simulink model "feeder_1_3_ss_pmu"  (Simulink 9.2)
settings: Solver=ode4  StartTime=0.0  StopTime=inf  FixedStep=0.0001  RelTol=1e-3
PreLoadFcn:
  | Ts=100e-6;Core_Num = 0;
PostLoadFcn:
  | Ts=100e-6;Core_Num = 0;
InitFcn:
  | Ts=100e-6;Core_Num = 0;
libraries: powerlib_meascontrol x153, rtio_generic_c37_118 x17, simulink x17, artemis x2, opal_lib x2, rtlab x1, powerlib x1
(part 2 of 4)

== system feeder_1_3_ss_pmu/SS_PMU/Subsystem9 ==
  Measurements : Inport
  Demux7 : Demux  Outputs=6
  Demux8 : Demux  Outputs=6
  Mux5 : Mux  Inputs=12
  Subsystem : Subsystem
  Phasors : Outport
  Phasor_Freq : Outport  Port=2
  FROC : Outport  Port=3
  wires:
  Mux5/1 -> Phasors/1
  Demux7/4 -> [Phase_Va]
  Demux7/1 -> [Mag_Va]
  Demux7/2 -> [Mag_Vb]
  Demux7/3 -> [Mag_Vc]
  Subsystem/1(Phasors_Vabc) -> Demux7/1
  Demux7/6 -> [Phase_Vc]
  Demux7/5 -> [Phase_Vb]
  Subsystem/3(Phasor_Freq) -> Phasor_Freq/1
  Measurements/1 -> Subsystem/1(Measurements1)
  Subsystem/4(Phasor_DTFreq) -> FROC/1
  Demux8/2 -> [Mag_Ib]
  Demux8/4 -> [Phase_Ia]
  Demux8/5 -> [Phase_Ib]
  Subsystem/2(Phasors_Iabc) -> Demux8/1
  Demux8/3 -> [Mag_Ic]
  Demux8/1 -> [Mag_Ia]
  Demux8/6 -> [Phase_Ic]
  [Phase_Ic] -> Mux5/12
  [Mag_Ic] -> Mux5/11
  [Phase_Ib] -> Mux5/10
  [Mag_Ib] -> Mux5/9
  [Phase_Ia] -> Mux5/8
  [Mag_Ia] -> Mux5/7
  [Phase_Vc] -> Mux5/6
  [Mag_Vc] -> Mux5/5
  [Phase_Vb] -> Mux5/4
  [Mag_Vb] -> Mux5/3
  [Phase_Va] -> Mux5/2
  [Mag_Va] -> Mux5/1

== system feeder_1_3_ss_pmu/SS_PMU/rtlab_send_subsystem ==

== system feeder_1_3_ss_pmu/SS_PMU/zzzOpComm ==
  Demux_1 : Demux  Outputs="[102    3   14]"
  Receive_1 : opal_lib/Communication/OpRec_rt  src=1  Data_width=119  st=0.0001
  busStruct : Subsystem
  Out1 : Outport
  Out2 : Outport  Port=2
  Out3 : Outport  Port=3
  wires:
  Demux_1/3 -> busStruct/3(In3)
  Demux_1/2 -> busStruct/2(In2)
  Demux_1/1 -> busStruct/1(In1)
  busStruct/3(Out3) -> Out3/1
  busStruct/2(Out2) -> Out2/1
  busStruct/1(Out1) -> Out1/1
  Receive_1/1 -> Demux_1/1

== system feeder_1_3_ss_pmu/SS_PMU/Subsystem1/Subsystem ==
  Measurements1 : Inport
  Demux7 : Demux  Outputs=2
  Subsystem1 : Subsystem
  Phasors_Vabc : Outport
  Phasors_Iabc : Outport  Port=2
  Phasor_Freq : Outport  Port=3
  Phasor_DTFreq : Outport  Port=4
  wires:
  Measurements1/1 -> Subsystem1/1(Measurements)
  Subsystem1/2(Phasors_Freq) -> Phasor_Freq/1
  Subsystem1/3(Phasors_DTFreq) -> Phasor_DTFreq/1
  Demux7/2 -> Phasors_Iabc/1
  Demux7/1 -> Phasors_Vabc/1
  Subsystem1/1(Phasors_abc) -> Demux7/1

== system feeder_1_3_ss_pmu/SS_PMU/Subsystem10/Subsystem ==
  Measurements1 : Inport
  Demux7 : Demux  Outputs=2
  Subsystem1 : Subsystem
  Phasors_Vabc : Outport
  Phasors_Iabc : Outport  Port=2
  Phasor_Freq : Outport  Port=3
  Phasor_DTFreq : Outport  Port=4
  wires:
  Measurements1/1 -> Subsystem1/1(Measurements)
  Subsystem1/2(Phasors_Freq) -> Phasor_Freq/1
  Subsystem1/3(Phasors_DTFreq) -> Phasor_DTFreq/1
  Demux7/2 -> Phasors_Iabc/1
  Demux7/1 -> Phasors_Vabc/1
  Subsystem1/1(Phasors_abc) -> Demux7/1

== system feeder_1_3_ss_pmu/SS_PMU/Subsystem11/Subsystem ==
  Measurements1 : Inport
  Demux7 : Demux  Outputs=2
  Subsystem1 : Subsystem
  Phasors_Vabc : Outport
  Phasors_Iabc : Outport  Port=2
  Phasor_Freq : Outport  Port=3
  Phasor_DTFreq : Outport  Port=4
  wires:
  Measurements1/1 -> Subsystem1/1(Measurements)
  Subsystem1/2(Phasors_Freq) -> Phasor_Freq/1
  Subsystem1/3(Phasors_DTFreq) -> Phasor_DTFreq/1
  Demux7/2 -> Phasors_Iabc/1
  Demux7/1 -> Phasors_Vabc/1
  Subsystem1/1(Phasors_abc) -> Demux7/1

== system feeder_1_3_ss_pmu/SS_PMU/Subsystem12/Subsystem ==
  Measurements1 : Inport
  Demux7 : Demux  Outputs=2
  Subsystem1 : Subsystem
  Phasors_Vabc : Outport
  Phasors_Iabc : Outport  Port=2
  Phasor_Freq : Outport  Port=3
  Phasor_DTFreq : Outport  Port=4
  wires:
  Measurements1/1 -> Subsystem1/1(Measurements)
  Subsystem1/2(Phasors_Freq) -> Phasor_Freq/1
  Subsystem1/3(Phasors_DTFreq) -> Phasor_DTFreq/1
  Demux7/2 -> Phasors_Iabc/1
  Demux7/1 -> Phasors_Vabc/1
  Subsystem1/1(Phasors_abc) -> Demux7/1

== system feeder_1_3_ss_pmu/SS_PMU/Subsystem13/Subsystem ==
  Measurements1 : Inport
  Demux7 : Demux  Outputs=2
  Subsystem1 : Subsystem
  Phasors_Vabc : Outport
  Phasors_Iabc : Outport  Port=2
  Phasor_Freq : Outport  Port=3
  Phasor_DTFreq : Outport  Port=4
  wires:
  Measurements1/1 -> Subsystem1/1(Measurements)
  Subsystem1/2(Phasors_Freq) -> Phasor_Freq/1
  Subsystem1/3(Phasors_DTFreq) -> Phasor_DTFreq/1
  Demux7/2 -> Phasors_Iabc/1
  Demux7/1 -> Phasors_Vabc/1
  Subsystem1/1(Phasors_abc) -> Demux7/1

== system feeder_1_3_ss_pmu/SS_PMU/Subsystem14/Subsystem ==
  Measurements1 : Inport
  Demux7 : Demux  Outputs=2
  Subsystem1 : Subsystem
  Phasors_Vabc : Outport
  Phasors_Iabc : Outport  Port=2
  Phasor_Freq : Outport  Port=3
  Phasor_DTFreq : Outport  Port=4
  wires:
  Measurements1/1 -> Subsystem1/1(Measurements)
  Subsystem1/2(Phasors_Freq) -> Phasor_Freq/1
  Subsystem1/3(Phasors_DTFreq) -> Phasor_DTFreq/1
  Demux7/2 -> Phasors_Iabc/1
  Demux7/1 -> Phasors_Vabc/1
  Subsystem1/1(Phasors_abc) -> Demux7/1

== system feeder_1_3_ss_pmu/SS_PMU/Subsystem15/Subsystem ==
  Measurements1 : Inport
  Demux7 : Demux  Outputs=2
  Subsystem1 : Subsystem
  Phasors_Vabc : Outport
  Phasors_Iabc : Outport  Port=2
  Phasor_Freq : Outport  Port=3
  Phasor_DTFreq : Outport  Port=4
  wires:
  Measurements1/1 -> Subsystem1/1(Measurements)
  Subsystem1/2(Phasors_Freq) -> Phasor_Freq/1
  Subsystem1/3(Phasors_DTFreq) -> Phasor_DTFreq/1
  Demux7/2 -> Phasors_Iabc/1
  Demux7/1 -> Phasors_Vabc/1
  Subsystem1/1(Phasors_abc) -> Demux7/1

== system feeder_1_3_ss_pmu/SS_PMU/Subsystem16/Subsystem ==
  Measurements1 : Inport
  Demux7 : Demux  Outputs=2
  Subsystem1 : Subsystem
  Phasors_Vabc : Outport
  Phasors_Iabc : Outport  Port=2
  Phasor_Freq : Outport  Port=3
  Phasor_DTFreq : Outport  Port=4
  wires:
  Measurements1/1 -> Subsystem1/1(Measurements)
  Subsystem1/2(Phasors_Freq) -> Phasor_Freq/1
  Subsystem1/3(Phasors_DTFreq) -> Phasor_DTFreq/1
  Demux7/2 -> Phasors_Iabc/1
  Demux7/1 -> Phasors_Vabc/1
  Subsystem1/1(Phasors_abc) -> Demux7/1

== system feeder_1_3_ss_pmu/SS_PMU/Subsystem17/Subsystem ==
  Measurements1 : Inport
  Demux7 : Demux  Outputs=2
  Subsystem1 : Subsystem
  Phasors_Vabc : Outport
  Phasors_Iabc : Outport  Port=2
  Phasor_Freq : Outport  Port=3
  Phasor_DTFreq : Outport  Port=4
  wires:
  Measurements1/1 -> Subsystem1/1(Measurements)
  Subsystem1/2(Phasors_Freq) -> Phasor_Freq/1
  Subsystem1/3(Phasors_DTFreq) -> Phasor_DTFreq/1
  Demux7/2 -> Phasors_Iabc/1
  Demux7/1 -> Phasors_Vabc/1
  Subsystem1/1(Phasors_abc) -> Demux7/1

== system feeder_1_3_ss_pmu/SS_PMU/Subsystem2/Subsystem ==
  Measurements1 : Inport
  Demux7 : Demux  Outputs=2
  Subsystem1 : Subsystem
  Phasors_Vabc : Outport
  Phasors_Iabc : Outport  Port=2
  Phasor_Freq : Outport  Port=3
  Phasor_DTFreq : Outport  Port=4
  wires:
  Measurements1/1 -> Subsystem1/1(Measurements)
  Subsystem1/2(Phasors_Freq) -> Phasor_Freq/1
  Subsystem1/3(Phasors_DTFreq) -> Phasor_DTFreq/1
  Demux7/2 -> Phasors_Iabc/1
  Demux7/1 -> Phasors_Vabc/1
  Subsystem1/1(Phasors_abc) -> Demux7/1

== system feeder_1_3_ss_pmu/SS_PMU/Subsystem20/Subsystem ==
  In1 : Inport
  Bus Creator : BusCreator  Inputs=3
  Selector1 : Selector  InputPortWidth=14  IndexOptions=Index vector (dialog)  Indices=[13]  OutputSizes=1
  Selector2 : Selector  InputPortWidth=14  IndexOptions=Index vector (dialog)  Indices=[14]  OutputSizes=1
  Selector5 : Selector  InputPortWidth=14  IndexOptions=Index vector (dialog)  Indices=[1 2 3 4 5 6 7 8 9 10 11 12]  OutputSizes=1
  Out1 : Outport
  wires:
  In1/1 -> Selector5/1, Selector2/1, Selector1/1
  Selector5/1 -> Bus Creator/1  "Measurements"
  Bus Creator/1 -> Out1/1
  Selector1/1 -> Bus Creator/2  "FREQ"
  Selector2/1 -> Bus Creator/3  "FROC"

== system feeder_1_3_ss_pmu/SS_PMU/Subsystem21/Subsystem ==
  In1 : Inport
  Bus Creator : BusCreator  Inputs=3
  Selector1 : Selector  InputPortWidth=14  IndexOptions=Index vector (dialog)  Indices=[13]  OutputSizes=1
  Selector2 : Selector  InputPortWidth=14  IndexOptions=Index vector (dialog)  Indices=[14]  OutputSizes=1
  Selector5 : Selector  InputPortWidth=14  IndexOptions=Index vector (dialog)  Indices=[1 2 3 4 5 6 7 8 9 10 11 12]  OutputSizes=1
  Out1 : Outport
  wires:
  In1/1 -> Selector5/1, Selector2/1, Selector1/1
  Selector5/1 -> Bus Creator/1  "Measurements"
  Bus Creator/1 -> Out1/1
  Selector1/1 -> Bus Creator/2  "FREQ"
  Selector2/1 -> Bus Creator/3  "FROC"

== system feeder_1_3_ss_pmu/SS_PMU/Subsystem24/Subsystem ==
  In1 : Inport
  Bus Creator : BusCreator  Inputs=3
  Selector1 : Selector  InputPortWidth=14  IndexOptions=Index vector (dialog)  Indices=[13]  OutputSizes=1
  Selector2 : Selector  InputPortWidth=14  IndexOptions=Index vector (dialog)  Indices=[14]  OutputSizes=1
  Selector5 : Selector  InputPortWidth=14  IndexOptions=Index vector (dialog)  Indices=[1 2 3 4 5 6 7 8 9 10 11 12]  OutputSizes=1
  Out1 : Outport
  wires:
  In1/1 -> Selector5/1, Selector2/1, Selector1/1
  Selector5/1 -> Bus Creator/1  "Measurements"
  Bus Creator/1 -> Out1/1
  Selector1/1 -> Bus Creator/2  "FREQ"
  Selector2/1 -> Bus Creator/3  "FROC"

== system feeder_1_3_ss_pmu/SS_PMU/Subsystem25/Subsystem ==
  In1 : Inport
  Bus Creator : BusCreator  Inputs=3
  Selector1 : Selector  InputPortWidth=14  IndexOptions=Index vector (dialog)  Indices=[13]  OutputSizes=1
  Selector2 : Selector  InputPortWidth=14  IndexOptions=Index vector (dialog)  Indices=[14]  OutputSizes=1
  Selector5 : Selector  InputPortWidth=14  IndexOptions=Index vector (dialog)  Indices=[1 2 3 4 5 6 7 8 9 10 11 12]  OutputSizes=1
  Out1 : Outport
  wires:
  In1/1 -> Selector5/1, Selector2/1, Selector1/1
  Selector5/1 -> Bus Creator/1  "Measurements"
  Bus Creator/1 -> Out1/1
  Selector1/1 -> Bus Creator/2  "FREQ"
  Selector2/1 -> Bus Creator/3  "FROC"

== system feeder_1_3_ss_pmu/SS_PMU/Subsystem26/Subsystem ==
  In1 : Inport
  Bus Creator : BusCreator  Inputs=3
  Selector1 : Selector  InputPortWidth=14  IndexOptions=Index vector (dialog)  Indices=[13]  OutputSizes=1
  Selector2 : Selector  InputPortWidth=14  IndexOptions=Index vector (dialog)  Indices=[14]  OutputSizes=1
  Selector5 : Selector  InputPortWidth=14  IndexOptions=Index vector (dialog)  Indices=[1 2 3 4 5 6 7 8 9 10 11 12]  OutputSizes=1
  Out1 : Outport
  wires:
  In1/1 -> Selector5/1, Selector2/1, Selector1/1
  Selector5/1 -> Bus Creator/1  "Measurements"
  Bus Creator/1 -> Out1/1
  Selector1/1 -> Bus Creator/2  "FREQ"
  Selector2/1 -> Bus Creator/3  "FROC"

== system feeder_1_3_ss_pmu/SS_PMU/Subsystem27/Subsystem ==
  In1 : Inport
  Bus Creator : BusCreator  Inputs=3
  Selector1 : Selector  InputPortWidth=14  IndexOptions=Index vector (dialog)  Indices=[13]  OutputSizes=1
  Selector2 : Selector  InputPortWidth=14  IndexOptions=Index vector (dialog)  Indices=[14]  OutputSizes=1
  Selector5 : Selector  InputPortWidth=14  IndexOptions=Index vector (dialog)  Indices=[1 2 3 4 5 6 7 8 9 10 11 12]  OutputSizes=1
  Out1 : Outport
  wires:
  In1/1 -> Selector5/1, Selector2/1, Selector1/1
  Selector5/1 -> Bus Creator/1  "Measurements"
  Bus Creator/1 -> Out1/1
  Selector1/1 -> Bus Creator/2  "FREQ"
  Selector2/1 -> Bus Creator/3  "FROC"

== system feeder_1_3_ss_pmu/SS_PMU/Subsystem28/Subsystem ==
  In1 : Inport
  Bus Creator : BusCreator  Inputs=3
  Selector1 : Selector  InputPortWidth=14  IndexOptions=Index vector (dialog)  Indices=[13]  OutputSizes=1
  Selector2 : Selector  InputPortWidth=14  IndexOptions=Index vector (dialog)  Indices=[14]  OutputSizes=1
  Selector5 : Selector  InputPortWidth=14  IndexOptions=Index vector (dialog)  Indices=[1 2 3 4 5 6 7 8 9 10 11 12]  OutputSizes=1
  Out1 : Outport
  wires:
  In1/1 -> Selector5/1, Selector2/1, Selector1/1
  Selector5/1 -> Bus Creator/1  "Measurements"
  Bus Creator/1 -> Out1/1
  Selector1/1 -> Bus Creator/2  "FREQ"
  Selector2/1 -> Bus Creator/3  "FROC"

== system feeder_1_3_ss_pmu/SS_PMU/Subsystem29/Subsystem ==
  In1 : Inport
  Bus Creator : BusCreator  Inputs=3
  Selector1 : Selector  InputPortWidth=14  IndexOptions=Index vector (dialog)  Indices=[13]  OutputSizes=1
  Selector2 : Selector  InputPortWidth=14  IndexOptions=Index vector (dialog)  Indices=[14]  OutputSizes=1
  Selector5 : Selector  InputPortWidth=14  IndexOptions=Index vector (dialog)  Indices=[1 2 3 4 5 6 7 8 9 10 11 12]  OutputSizes=1
  Out1 : Outport
  wires:
  In1/1 -> Selector5/1, Selector2/1, Selector1/1
  Selector5/1 -> Bus Creator/1  "Measurements"
  Bus Creator/1 -> Out1/1
  Selector1/1 -> Bus Creator/2  "FREQ"
  Selector2/1 -> Bus Creator/3  "FROC"

== system feeder_1_3_ss_pmu/SS_PMU/Subsystem3/Subsystem ==
  Measurements1 : Inport
  Demux7 : Demux  Outputs=2
  Subsystem1 : Subsystem
  Phasors_Vabc : Outport
  Phasors_Iabc : Outport  Port=2
  Phasor_Freq : Outport  Port=3
  Phasor_DTFreq : Outport  Port=4
  wires:
  Measurements1/1 -> Subsystem1/1(Measurements)
  Subsystem1/2(Phasors_Freq) -> Phasor_Freq/1
  Subsystem1/3(Phasors_DTFreq) -> Phasor_DTFreq/1
  Demux7/2 -> Phasors_Iabc/1
  Demux7/1 -> Phasors_Vabc/1
  Subsystem1/1(Phasors_abc) -> Demux7/1

== system feeder_1_3_ss_pmu/SS_PMU/Subsystem30/Subsystem ==
  In1 : Inport
  Bus Creator : BusCreator  Inputs=3
  Selector1 : Selector  InputPortWidth=14  IndexOptions=Index vector (dialog)  Indices=[13]  OutputSizes=1
  Selector2 : Selector  InputPortWidth=14  IndexOptions=Index vector (dialog)  Indices=[14]  OutputSizes=1
  Selector5 : Selector  InputPortWidth=14  IndexOptions=Index vector (dialog)  Indices=[1 2 3 4 5 6 7 8 9 10 11 12]  OutputSizes=1
  Out1 : Outport
  wires:
  In1/1 -> Selector5/1, Selector2/1, Selector1/1
  Selector5/1 -> Bus Creator/1  "Measurements"
  Bus Creator/1 -> Out1/1
  Selector1/1 -> Bus Creator/2  "FREQ"
  Selector2/1 -> Bus Creator/3  "FROC"

== system feeder_1_3_ss_pmu/SS_PMU/Subsystem31/Subsystem ==
  In1 : Inport
  Bus Creator : BusCreator  Inputs=3
  Selector1 : Selector  InputPortWidth=14  IndexOptions=Index vector (dialog)  Indices=[13]  OutputSizes=1
  Selector2 : Selector  InputPortWidth=14  IndexOptions=Index vector (dialog)  Indices=[14]  OutputSizes=1
  Selector5 : Selector  InputPortWidth=14  IndexOptions=Index vector (dialog)  Indices=[1 2 3 4 5 6 7 8 9 10 11 12]  OutputSizes=1
  Out1 : Outport
  wires:
  In1/1 -> Selector5/1, Selector2/1, Selector1/1
  Selector5/1 -> Bus Creator/1  "Measurements"
  Bus Creator/1 -> Out1/1
  Selector1/1 -> Bus Creator/2  "FREQ"
  Selector2/1 -> Bus Creator/3  "FROC"

== system feeder_1_3_ss_pmu/SS_PMU/Subsystem32/Subsystem ==
  In1 : Inport
  Bus Creator : BusCreator  Inputs=3
  Selector1 : Selector  InputPortWidth=14  IndexOptions=Index vector (dialog)  Indices=[13]  OutputSizes=1
  Selector2 : Selector  InputPortWidth=14  IndexOptions=Index vector (dialog)  Indices=[14]  OutputSizes=1
  Selector5 : Selector  InputPortWidth=14  IndexOptions=Index vector (dialog)  Indices=[1 2 3 4 5 6 7 8 9 10 11 12]  OutputSizes=1
  Out1 : Outport
  wires:
  In1/1 -> Selector5/1, Selector2/1, Selector1/1
  Selector5/1 -> Bus Creator/1  "Measurements"
  Bus Creator/1 -> Out1/1
  Selector1/1 -> Bus Creator/2  "FREQ"
  Selector2/1 -> Bus Creator/3  "FROC"

== system feeder_1_3_ss_pmu/SS_PMU/Subsystem33/Subsystem ==
  In1 : Inport
  Bus Creator : BusCreator  Inputs=3
  Selector1 : Selector  InputPortWidth=14  IndexOptions=Index vector (dialog)  Indices=[13]  OutputSizes=1
  Selector2 : Selector  InputPortWidth=14  IndexOptions=Index vector (dialog)  Indices=[14]  OutputSizes=1
  Selector5 : Selector  InputPortWidth=14  IndexOptions=Index vector (dialog)  Indices=[1 2 3 4 5 6 7 8 9 10 11 12]  OutputSizes=1
  Out1 : Outport
  wires:
  In1/1 -> Selector5/1, Selector2/1, Selector1/1
  Selector5/1 -> Bus Creator/1  "Measurements"
  Bus Creator/1 -> Out1/1
  Selector1/1 -> Bus Creator/2  "FREQ"
  Selector2/1 -> Bus Creator/3  "FROC"

== system feeder_1_3_ss_pmu/SS_PMU/Subsystem34/Subsystem ==
  In1 : Inport
  Bus Creator : BusCreator  Inputs=3
  Selector1 : Selector  InputPortWidth=14  IndexOptions=Index vector (dialog)  Indices=[13]  OutputSizes=1
  Selector2 : Selector  InputPortWidth=14  IndexOptions=Index vector (dialog)  Indices=[14]  OutputSizes=1
  Selector5 : Selector  InputPortWidth=14  IndexOptions=Index vector (dialog)  Indices=[1 2 3 4 5 6 7 8 9 10 11 12]  OutputSizes=1
  Out1 : Outport
  wires:
  In1/1 -> Selector5/1, Selector2/1, Selector1/1
  Selector5/1 -> Bus Creator/1  "Measurements"
  Bus Creator/1 -> Out1/1
  Selector1/1 -> Bus Creator/2  "FREQ"
  Selector2/1 -> Bus Creator/3  "FROC"

== system feeder_1_3_ss_pmu/SS_PMU/Subsystem35/Subsystem ==
  In1 : Inport
  Bus Creator : BusCreator  Inputs=3
  Selector1 : Selector  InputPortWidth=14  IndexOptions=Index vector (dialog)  Indices=[13]  OutputSizes=1
  Selector2 : Selector  InputPortWidth=14  IndexOptions=Index vector (dialog)  Indices=[14]  OutputSizes=1
  Selector5 : Selector  InputPortWidth=14  IndexOptions=Index vector (dialog)  Indices=[1 2 3 4 5 6 7 8 9 10 11 12]  OutputSizes=1
  Out1 : Outport
  wires:
  In1/1 -> Selector5/1, Selector2/1, Selector1/1
  Selector5/1 -> Bus Creator/1  "Measurements"
  Bus Creator/1 -> Out1/1
  Selector1/1 -> Bus Creator/2  "FREQ"
  Selector2/1 -> Bus Creator/3  "FROC"

== system feeder_1_3_ss_pmu/SS_PMU/Subsystem36/Subsystem ==
  In1 : Inport
  Bus Creator : BusCreator  Inputs=3
  Selector1 : Selector  InputPortWidth=14  IndexOptions=Index vector (dialog)  Indices=[13]  OutputSizes=1
  Selector2 : Selector  InputPortWidth=14  IndexOptions=Index vector (dialog)  Indices=[14]  OutputSizes=1
  Selector5 : Selector  InputPortWidth=14  IndexOptions=Index vector (dialog)  Indices=[1 2 3 4 5 6 7 8 9 10 11 12]  OutputSizes=1
  Out1 : Outport
  wires:
  In1/1 -> Selector5/1, Selector2/1, Selector1/1
  Selector5/1 -> Bus Creator/1  "Measurements"
  Bus Creator/1 -> Out1/1
  Selector1/1 -> Bus Creator/2  "FREQ"
  Selector2/1 -> Bus Creator/3  "FROC"

== system feeder_1_3_ss_pmu/SS_PMU/Subsystem37/Subsystem ==
  In1 : Inport
  Bus Creator : BusCreator  Inputs=3
  Selector1 : Selector  InputPortWidth=14  IndexOptions=Index vector (dialog)  Indices=[13]  OutputSizes=1
  Selector2 : Selector  InputPortWidth=14  IndexOptions=Index vector (dialog)  Indices=[14]  OutputSizes=1
  Selector5 : Selector  InputPortWidth=14  IndexOptions=Index vector (dialog)  Indices=[1 2 3 4 5 6 7 8 9 10 11 12]  OutputSizes=1
  Out1 : Outport
  wires:
  In1/1 -> Selector5/1, Selector2/1, Selector1/1
  Selector5/1 -> Bus Creator/1  "Measurements"
  Bus Creator/1 -> Out1/1
  Selector1/1 -> Bus Creator/2  "FREQ"
  Selector2/1 -> Bus Creator/3  "FROC"

== system feeder_1_3_ss_pmu/SS_PMU/Subsystem38/Subsystem ==
  In1 : Inport
  Bus Creator : BusCreator  Inputs=3
  Selector1 : Selector  InputPortWidth=14  IndexOptions=Index vector (dialog)  Indices=[13]  OutputSizes=1
  Selector2 : Selector  InputPortWidth=14  IndexOptions=Index vector (dialog)  Indices=[14]  OutputSizes=1
  Selector5 : Selector  InputPortWidth=14  IndexOptions=Index vector (dialog)  Indices=[1 2 3 4 5 6 7 8 9 10 11 12]  OutputSizes=1
  Out1 : Outport
  wires:
  In1/1 -> Selector5/1, Selector2/1, Selector1/1
  Selector5/1 -> Bus Creator/1  "Measurements"
  Bus Creator/1 -> Out1/1
  Selector1/1 -> Bus Creator/2  "FREQ"
  Selector2/1 -> Bus Creator/3  "FROC"

== system feeder_1_3_ss_pmu/SS_PMU/Subsystem4/Subsystem ==
  Measurements1 : Inport
  Demux7 : Demux  Outputs=2
  Subsystem1 : Subsystem
  Phasors_Vabc : Outport
  Phasors_Iabc : Outport  Port=2
  Phasor_Freq : Outport  Port=3
  Phasor_DTFreq : Outport  Port=4
  wires:
  Measurements1/1 -> Subsystem1/1(Measurements)
  Subsystem1/2(Phasors_Freq) -> Phasor_Freq/1
  Subsystem1/3(Phasors_DTFreq) -> Phasor_DTFreq/1
  Demux7/2 -> Phasors_Iabc/1
  Demux7/1 -> Phasors_Vabc/1
  Subsystem1/1(Phasors_abc) -> Demux7/1

== system feeder_1_3_ss_pmu/SS_PMU/Subsystem5/Subsystem ==
  Measurements1 : Inport
  Demux7 : Demux  Outputs=2
  Subsystem1 : Subsystem
  Phasors_Vabc : Outport
  Phasors_Iabc : Outport  Port=2
  Phasor_Freq : Outport  Port=3
  Phasor_DTFreq : Outport  Port=4
  wires:
  Measurements1/1 -> Subsystem1/1(Measurements)
  Subsystem1/2(Phasors_Freq) -> Phasor_Freq/1
  Subsystem1/3(Phasors_DTFreq) -> Phasor_DTFreq/1
  Demux7/2 -> Phasors_Iabc/1
  Demux7/1 -> Phasors_Vabc/1
  Subsystem1/1(Phasors_abc) -> Demux7/1

== system feeder_1_3_ss_pmu/SS_PMU/Subsystem6/Subsystem ==
  Measurements1 : Inport
  Demux7 : Demux  Outputs=2
  Subsystem1 : Subsystem
  Phasors_Vabc : Outport
  Phasors_Iabc : Outport  Port=2
  Phasor_Freq : Outport  Port=3
  Phasor_DTFreq : Outport  Port=4
  wires:
  Measurements1/1 -> Subsystem1/1(Measurements)
  Subsystem1/2(Phasors_Freq) -> Phasor_Freq/1
  Subsystem1/3(Phasors_DTFreq) -> Phasor_DTFreq/1
  Demux7/2 -> Phasors_Iabc/1
  Demux7/1 -> Phasors_Vabc/1
  Subsystem1/1(Phasors_abc) -> Demux7/1

== system feeder_1_3_ss_pmu/SS_PMU/Subsystem7/Subsystem ==
  Measurements1 : Inport
  Demux7 : Demux  Outputs=2
  Subsystem1 : Subsystem
  Phasors_Vabc : Outport
  Phasors_Iabc : Outport  Port=2
  Phasor_Freq : Outport  Port=3
  Phasor_DTFreq : Outport  Port=4
  wires:
  Measurements1/1 -> Subsystem1/1(Measurements)
  Subsystem1/2(Phasors_Freq) -> Phasor_Freq/1
  Subsystem1/3(Phasors_DTFreq) -> Phasor_DTFreq/1
  Demux7/2 -> Phasors_Iabc/1
  Demux7/1 -> Phasors_Vabc/1
  Subsystem1/1(Phasors_abc) -> Demux7/1

== system feeder_1_3_ss_pmu/SS_PMU/Subsystem8/Subsystem ==
  Measurements1 : Inport
  Demux7 : Demux  Outputs=2
  Subsystem1 : Subsystem
  Phasors_Vabc : Outport
  Phasors_Iabc : Outport  Port=2
  Phasor_Freq : Outport  Port=3
  Phasor_DTFreq : Outport  Port=4
  wires:
  Measurements1/1 -> Subsystem1/1(Measurements)
  Subsystem1/2(Phasors_Freq) -> Phasor_Freq/1
  Subsystem1/3(Phasors_DTFreq) -> Phasor_DTFreq/1
  Demux7/2 -> Phasors_Iabc/1
  Demux7/1 -> Phasors_Vabc/1
  Subsystem1/1(Phasors_abc) -> Demux7/1

== system feeder_1_3_ss_pmu/SS_PMU/Subsystem9/Subsystem ==
  Measurements1 : Inport
  Demux7 : Demux  Outputs=2
  Subsystem1 : Subsystem
  Phasors_Vabc : Outport
  Phasors_Iabc : Outport  Port=2
  Phasor_Freq : Outport  Port=3
  Phasor_DTFreq : Outport  Port=4
  wires:
  Measurements1/1 -> Subsystem1/1(Measurements)
  Subsystem1/2(Phasors_Freq) -> Phasor_Freq/1
  Subsystem1/3(Phasors_DTFreq) -> Phasor_DTFreq/1
  Demux7/2 -> Phasors_Iabc/1
  Demux7/1 -> Phasors_Vabc/1
  Subsystem1/1(Phasors_abc) -> Demux7/1

== system feeder_1_3_ss_pmu/SS_PMU/zzzOpComm/busStruct ==
  In1 : Inport
  In2 : Inport  Port=2
  In3 : Inport  Port=3
  Sub1 : Subsystem
  Sub2 : Subsystem
  Sub3 : Subsystem
  Out1 : Outport
  Out2 : Outport  Port=2
  Out3 : Outport  Port=3
  wires:
  Sub3/1(out) -> Out3/1
  In3/1 -> Sub3/1(in)
  Sub2/1(out) -> Out2/1
  In2/1 -> Sub2/1(in)
  Sub1/1(goto_signal1) -> Out1/1
  In1/1 -> Sub1/1(from_signal1)

== system feeder_1_3_ss_pmu/SS_PMU/Subsystem1/Subsystem/Subsystem1 ==
  Measurements : Inport
  Degree to radian1 : Subsystem
  Mux1 : Mux
  Selector5 : Selector  InputPortWidth=12  IndexOptions=Index vector (dialog)  Indices=[1 3 5]  OutputSizes=1
  Selector6 : Selector  InputPortWidth=12  IndexOptions=Index vector (dialog)  Indices=[7 9 11]  OutputSizes=1
  Selector7 : Selector  InputPortWidth=6  IndexOptions=Index vector (dialog)  Indices=[1 2 3]  OutputSizes=1
  Selector8 : Selector  InputPortWidth=6  IndexOptions=Index vector (dialog)  Indices=[4 5 6]  OutputSizes=1
  Selector9 : Selector  InputPortWidth=12  IndexOptions=Index vector (dialog)  Indices=[2 4 6 8 10 12]  OutputSizes=1
  Subsystem : Subsystem
  Phasors_abc : Outport
  Phasors_Freq : Outport  Port=2
  Phasors_DTFreq : Outport  Port=3
  wires:
  Subsystem/2(Phasors_freq) -> Phasors_Freq/1
  Subsystem/3(Phasors_dtfreq1) -> Phasors_DTFreq/1
  Selector5/1 -> Mux1/1
  Mux1/1 -> Phasors_abc/1
  Selector7/1 -> Mux1/2
  Subsystem/1(Phasors_60Hz) -> Selector5/1, Selector6/1, Selector9/1
  Selector8/1 -> Mux1/4
  Selector6/1 -> Mux1/3
  Measurements/1 -> Subsystem/1(Measurements1)
  Selector9/1 -> Degree to radian1/1(Degree)
  Degree to radian1/1(Radian) -> Selector7/1, Selector8/1

== system feeder_1_3_ss_pmu/SS_PMU/Subsystem10/Subsystem/Subsystem1 ==
  Measurements : Inport
  Degree to radian1 : Subsystem
  Mux1 : Mux
  Selector5 : Selector  InputPortWidth=12  IndexOptions=Index vector (dialog)  Indices=[1 3 5]  OutputSizes=1
  Selector6 : Selector  InputPortWidth=12  IndexOptions=Index vector (dialog)  Indices=[7 9 11]  OutputSizes=1
  Selector7 : Selector  InputPortWidth=6  IndexOptions=Index vector (dialog)  Indices=[1 2 3]  OutputSizes=1
  Selector8 : Selector  InputPortWidth=6  IndexOptions=Index vector (dialog)  Indices=[4 5 6]  OutputSizes=1
  Selector9 : Selector  InputPortWidth=12  IndexOptions=Index vector (dialog)  Indices=[2 4 6 8 10 12]  OutputSizes=1
  Subsystem : Subsystem
  Phasors_abc : Outport
  Phasors_Freq : Outport  Port=2
  Phasors_DTFreq : Outport  Port=3
  wires:
  Subsystem/2(Phasors_freq) -> Phasors_Freq/1
  Subsystem/3(Phasors_dtfreq1) -> Phasors_DTFreq/1
  Selector5/1 -> Mux1/1
  Mux1/1 -> Phasors_abc/1
  Selector7/1 -> Mux1/2
  Subsystem/1(Phasors_60Hz) -> Selector5/1, Selector6/1, Selector9/1
  Selector8/1 -> Mux1/4
  Selector6/1 -> Mux1/3
  Measurements/1 -> Subsystem/1(Measurements1)
  Selector9/1 -> Degree to radian1/1(Degree)
  Degree to radian1/1(Radian) -> Selector7/1, Selector8/1

== system feeder_1_3_ss_pmu/SS_PMU/Subsystem11/Subsystem/Subsystem1 ==
  Measurements : Inport
  Degree to radian1 : Subsystem
  Mux1 : Mux
  Selector5 : Selector  InputPortWidth=12  IndexOptions=Index vector (dialog)  Indices=[1 3 5]  OutputSizes=1
  Selector6 : Selector  InputPortWidth=12  IndexOptions=Index vector (dialog)  Indices=[7 9 11]  OutputSizes=1
  Selector7 : Selector  InputPortWidth=6  IndexOptions=Index vector (dialog)  Indices=[1 2 3]  OutputSizes=1
  Selector8 : Selector  InputPortWidth=6  IndexOptions=Index vector (dialog)  Indices=[4 5 6]  OutputSizes=1
  Selector9 : Selector  InputPortWidth=12  IndexOptions=Index vector (dialog)  Indices=[2 4 6 8 10 12]  OutputSizes=1
  Subsystem : Subsystem
  Phasors_abc : Outport
  Phasors_Freq : Outport  Port=2
  Phasors_DTFreq : Outport  Port=3
  wires:
  Subsystem/2(Phasors_freq) -> Phasors_Freq/1
  Subsystem/3(Phasors_dtfreq1) -> Phasors_DTFreq/1
  Selector5/1 -> Mux1/1
  Mux1/1 -> Phasors_abc/1
  Selector7/1 -> Mux1/2
  Subsystem/1(Phasors_60Hz) -> Selector5/1, Selector6/1, Selector9/1
  Selector8/1 -> Mux1/4
  Selector6/1 -> Mux1/3
  Measurements/1 -> Subsystem/1(Measurements1)
  Selector9/1 -> Degree to radian1/1(Degree)
  Degree to radian1/1(Radian) -> Selector7/1, Selector8/1

== system feeder_1_3_ss_pmu/SS_PMU/Subsystem12/Subsystem/Subsystem1 ==
  Measurements : Inport
  Degree to radian1 : Subsystem
  Mux1 : Mux
  Selector5 : Selector  InputPortWidth=12  IndexOptions=Index vector (dialog)  Indices=[1 3 5]  OutputSizes=1
  Selector6 : Selector  InputPortWidth=12  IndexOptions=Index vector (dialog)  Indices=[7 9 11]  OutputSizes=1
  Selector7 : Selector  InputPortWidth=6  IndexOptions=Index vector (dialog)  Indices=[1 2 3]  OutputSizes=1
  Selector8 : Selector  InputPortWidth=6  IndexOptions=Index vector (dialog)  Indices=[4 5 6]  OutputSizes=1
  Selector9 : Selector  InputPortWidth=12  IndexOptions=Index vector (dialog)  Indices=[2 4 6 8 10 12]  OutputSizes=1
  Subsystem : Subsystem
  Phasors_abc : Outport
  Phasors_Freq : Outport  Port=2
  Phasors_DTFreq : Outport  Port=3
  wires:
  Subsystem/2(Phasors_freq) -> Phasors_Freq/1
  Subsystem/3(Phasors_dtfreq1) -> Phasors_DTFreq/1
  Selector5/1 -> Mux1/1
  Mux1/1 -> Phasors_abc/1
  Selector7/1 -> Mux1/2
  Subsystem/1(Phasors_60Hz) -> Selector5/1, Selector6/1, Selector9/1
  Selector8/1 -> Mux1/4
  Selector6/1 -> Mux1/3
  Measurements/1 -> Subsystem/1(Measurements1)
  Selector9/1 -> Degree to radian1/1(Degree)
  Degree to radian1/1(Radian) -> Selector7/1, Selector8/1

== system feeder_1_3_ss_pmu/SS_PMU/Subsystem13/Subsystem/Subsystem1 ==
  Measurements : Inport
  Degree to radian1 : Subsystem
  Mux1 : Mux
  Selector5 : Selector  InputPortWidth=12  IndexOptions=Index vector (dialog)  Indices=[1 3 5]  OutputSizes=1
  Selector6 : Selector  InputPortWidth=12  IndexOptions=Index vector (dialog)  Indices=[7 9 11]  OutputSizes=1
  Selector7 : Selector  InputPortWidth=6  IndexOptions=Index vector (dialog)  Indices=[1 2 3]  OutputSizes=1
  Selector8 : Selector  InputPortWidth=6  IndexOptions=Index vector (dialog)  Indices=[4 5 6]  OutputSizes=1
  Selector9 : Selector  InputPortWidth=12  IndexOptions=Index vector (dialog)  Indices=[2 4 6 8 10 12]  OutputSizes=1
  Subsystem : Subsystem
  Phasors_abc : Outport
  Phasors_Freq : Outport  Port=2
  Phasors_DTFreq : Outport  Port=3
  wires:
  Subsystem/2(Phasors_freq) -> Phasors_Freq/1
  Subsystem/3(Phasors_dtfreq1) -> Phasors_DTFreq/1
  Selector5/1 -> Mux1/1
  Mux1/1 -> Phasors_abc/1
  Selector7/1 -> Mux1/2
  Subsystem/1(Phasors_60Hz) -> Selector5/1, Selector6/1, Selector9/1
  Selector8/1 -> Mux1/4
  Selector6/1 -> Mux1/3
  Measurements/1 -> Subsystem/1(Measurements1)
  Selector9/1 -> Degree to radian1/1(Degree)
  Degree to radian1/1(Radian) -> Selector7/1, Selector8/1

== system feeder_1_3_ss_pmu/SS_PMU/Subsystem14/Subsystem/Subsystem1 ==
  Measurements : Inport
  Degree to radian1 : Subsystem
  Mux1 : Mux
  Selector5 : Selector  InputPortWidth=12  IndexOptions=Index vector (dialog)  Indices=[1 3 5]  OutputSizes=1
  Selector6 : Selector  InputPortWidth=12  IndexOptions=Index vector (dialog)  Indices=[7 9 11]  OutputSizes=1
  Selector7 : Selector  InputPortWidth=6  IndexOptions=Index vector (dialog)  Indices=[1 2 3]  OutputSizes=1
  Selector8 : Selector  InputPortWidth=6  IndexOptions=Index vector (dialog)  Indices=[4 5 6]  OutputSizes=1
  Selector9 : Selector  InputPortWidth=12  IndexOptions=Index vector (dialog)  Indices=[2 4 6 8 10 12]  OutputSizes=1
  Subsystem : Subsystem
  Phasors_abc : Outport
  Phasors_Freq : Outport  Port=2
  Phasors_DTFreq : Outport  Port=3
  wires:
  Subsystem/2(Phasors_freq) -> Phasors_Freq/1
  Subsystem/3(Phasors_dtfreq1) -> Phasors_DTFreq/1
  Selector5/1 -> Mux1/1
  Mux1/1 -> Phasors_abc/1
  Selector7/1 -> Mux1/2
  Subsystem/1(Phasors_60Hz) -> Selector5/1, Selector6/1, Selector9/1
  Selector8/1 -> Mux1/4
  Selector6/1 -> Mux1/3
  Measurements/1 -> Subsystem/1(Measurements1)
  Selector9/1 -> Degree to radian1/1(Degree)
  Degree to radian1/1(Radian) -> Selector7/1, Selector8/1

== system feeder_1_3_ss_pmu/SS_PMU/Subsystem15/Subsystem/Subsystem1 ==
  Measurements : Inport
  Degree to radian1 : Subsystem
  Mux1 : Mux
  Selector5 : Selector  InputPortWidth=12  IndexOptions=Index vector (dialog)  Indices=[1 3 5]  OutputSizes=1
  Selector6 : Selector  InputPortWidth=12  IndexOptions=Index vector (dialog)  Indices=[7 9 11]  OutputSizes=1
  Selector7 : Selector  InputPortWidth=6  IndexOptions=Index vector (dialog)  Indices=[1 2 3]  OutputSizes=1
  Selector8 : Selector  InputPortWidth=6  IndexOptions=Index vector (dialog)  Indices=[4 5 6]  OutputSizes=1
  Selector9 : Selector  InputPortWidth=12  IndexOptions=Index vector (dialog)  Indices=[2 4 6 8 10 12]  OutputSizes=1
  Subsystem : Subsystem
  Phasors_abc : Outport
  Phasors_Freq : Outport  Port=2
  Phasors_DTFreq : Outport  Port=3
  wires:
  Subsystem/2(Phasors_freq) -> Phasors_Freq/1
  Subsystem/3(Phasors_dtfreq1) -> Phasors_DTFreq/1
  Selector5/1 -> Mux1/1
  Mux1/1 -> Phasors_abc/1
  Selector7/1 -> Mux1/2
  Subsystem/1(Phasors_60Hz) -> Selector5/1, Selector6/1, Selector9/1
  Selector8/1 -> Mux1/4
  Selector6/1 -> Mux1/3
  Measurements/1 -> Subsystem/1(Measurements1)
  Selector9/1 -> Degree to radian1/1(Degree)
  Degree to radian1/1(Radian) -> Selector7/1, Selector8/1

== system feeder_1_3_ss_pmu/SS_PMU/Subsystem16/Subsystem/Subsystem1 ==
  Measurements : Inport
  Degree to radian1 : Subsystem
  Mux1 : Mux
  Selector5 : Selector  InputPortWidth=12  IndexOptions=Index vector (dialog)  Indices=[1 3 5]  OutputSizes=1
  Selector6 : Selector  InputPortWidth=12  IndexOptions=Index vector (dialog)  Indices=[7 9 11]  OutputSizes=1
  Selector7 : Selector  InputPortWidth=6  IndexOptions=Index vector (dialog)  Indices=[1 2 3]  OutputSizes=1
  Selector8 : Selector  InputPortWidth=6  IndexOptions=Index vector (dialog)  Indices=[4 5 6]  OutputSizes=1
  Selector9 : Selector  InputPortWidth=12  IndexOptions=Index vector (dialog)  Indices=[2 4 6 8 10 12]  OutputSizes=1
  Subsystem : Subsystem
  Phasors_abc : Outport
  Phasors_Freq : Outport  Port=2
  Phasors_DTFreq : Outport  Port=3
  wires:
  Subsystem/2(Phasors_freq) -> Phasors_Freq/1
  Subsystem/3(Phasors_dtfreq1) -> Phasors_DTFreq/1
  Selector5/1 -> Mux1/1
  Mux1/1 -> Phasors_abc/1
  Selector7/1 -> Mux1/2
  Subsystem/1(Phasors_60Hz) -> Selector5/1, Selector6/1, Selector9/1
  Selector8/1 -> Mux1/4
  Selector6/1 -> Mux1/3
  Measurements/1 -> Subsystem/1(Measurements1)
  Selector9/1 -> Degree to radian1/1(Degree)
  Degree to radian1/1(Radian) -> Selector7/1, Selector8/1

== system feeder_1_3_ss_pmu/SS_PMU/Subsystem17/Subsystem/Subsystem1 ==
  Measurements : Inport
  Degree to radian1 : Subsystem
  Mux1 : Mux
  Selector5 : Selector  InputPortWidth=12  IndexOptions=Index vector (dialog)  Indices=[1 3 5]  OutputSizes=1
  Selector6 : Selector  InputPortWidth=12  IndexOptions=Index vector (dialog)  Indices=[7 9 11]  OutputSizes=1
  Selector7 : Selector  InputPortWidth=6  IndexOptions=Index vector (dialog)  Indices=[1 2 3]  OutputSizes=1
  Selector8 : Selector  InputPortWidth=6  IndexOptions=Index vector (dialog)  Indices=[4 5 6]  OutputSizes=1
  Selector9 : Selector  InputPortWidth=12  IndexOptions=Index vector (dialog)  Indices=[2 4 6 8 10 12]  OutputSizes=1
  Subsystem : Subsystem
  Phasors_abc : Outport
  Phasors_Freq : Outport  Port=2
  Phasors_DTFreq : Outport  Port=3
  wires:
  Subsystem/2(Phasors_freq) -> Phasors_Freq/1
  Subsystem/3(Phasors_dtfreq1) -> Phasors_DTFreq/1
  Selector5/1 -> Mux1/1
  Mux1/1 -> Phasors_abc/1
  Selector7/1 -> Mux1/2
  Subsystem/1(Phasors_60Hz) -> Selector5/1, Selector6/1, Selector9/1
  Selector8/1 -> Mux1/4
  Selector6/1 -> Mux1/3
  Measurements/1 -> Subsystem/1(Measurements1)
  Selector9/1 -> Degree to radian1/1(Degree)
  Degree to radian1/1(Radian) -> Selector7/1, Selector8/1

== system feeder_1_3_ss_pmu/SS_PMU/Subsystem2/Subsystem/Subsystem1 ==
  Measurements : Inport
  Degree to radian1 : Subsystem
  Mux1 : Mux
  Selector5 : Selector  InputPortWidth=12  IndexOptions=Index vector (dialog)  Indices=[1 3 5]  OutputSizes=1
  Selector6 : Selector  InputPortWidth=12  IndexOptions=Index vector (dialog)  Indices=[7 9 11]  OutputSizes=1
  Selector7 : Selector  InputPortWidth=6  IndexOptions=Index vector (dialog)  Indices=[1 2 3]  OutputSizes=1
  Selector8 : Selector  InputPortWidth=6  IndexOptions=Index vector (dialog)  Indices=[4 5 6]  OutputSizes=1
  Selector9 : Selector  InputPortWidth=12  IndexOptions=Index vector (dialog)  Indices=[2 4 6 8 10 12]  OutputSizes=1
  Subsystem : Subsystem
  Phasors_abc : Outport
  Phasors_Freq : Outport  Port=2
  Phasors_DTFreq : Outport  Port=3
  wires:
  Subsystem/2(Phasors_freq) -> Phasors_Freq/1
  Subsystem/3(Phasors_dtfreq1) -> Phasors_DTFreq/1
  Selector5/1 -> Mux1/1
  Mux1/1 -> Phasors_abc/1
  Selector7/1 -> Mux1/2
  Subsystem/1(Phasors_60Hz) -> Selector5/1, Selector6/1, Selector9/1
  Selector8/1 -> Mux1/4
  Selector6/1 -> Mux1/3
  Measurements/1 -> Subsystem/1(Measurements1)
  Selector9/1 -> Degree to radian1/1(Degree)
  Degree to radian1/1(Radian) -> Selector7/1, Selector8/1

== system feeder_1_3_ss_pmu/SS_PMU/Subsystem3/Subsystem/Subsystem1 ==
  Measurements : Inport
  Degree to radian1 : Subsystem
  Mux1 : Mux
  Selector5 : Selector  InputPortWidth=12  IndexOptions=Index vector (dialog)  Indices=[1 3 5]  OutputSizes=1
  Selector6 : Selector  InputPortWidth=12  IndexOptions=Index vector (dialog)  Indices=[7 9 11]  OutputSizes=1
  Selector7 : Selector  InputPortWidth=6  IndexOptions=Index vector (dialog)  Indices=[1 2 3]  OutputSizes=1
  Selector8 : Selector  InputPortWidth=6  IndexOptions=Index vector (dialog)  Indices=[4 5 6]  OutputSizes=1
  Selector9 : Selector  InputPortWidth=12  IndexOptions=Index vector (dialog)  Indices=[2 4 6 8 10 12]  OutputSizes=1
  Subsystem : Subsystem
  Phasors_abc : Outport
  Phasors_Freq : Outport  Port=2
  Phasors_DTFreq : Outport  Port=3
  wires:
  Subsystem/2(Phasors_freq) -> Phasors_Freq/1
  Subsystem/3(Phasors_dtfreq1) -> Phasors_DTFreq/1
  Selector5/1 -> Mux1/1
  Mux1/1 -> Phasors_abc/1
  Selector7/1 -> Mux1/2
  Subsystem/1(Phasors_60Hz) -> Selector5/1, Selector6/1, Selector9/1
  Selector8/1 -> Mux1/4
  Selector6/1 -> Mux1/3
  Measurements/1 -> Subsystem/1(Measurements1)
  Selector9/1 -> Degree to radian1/1(Degree)
  Degree to radian1/1(Radian) -> Selector7/1, Selector8/1

== system feeder_1_3_ss_pmu/SS_PMU/Subsystem4/Subsystem/Subsystem1 ==
  Measurements : Inport
  Degree to radian1 : Subsystem
  Mux1 : Mux
  Selector5 : Selector  InputPortWidth=12  IndexOptions=Index vector (dialog)  Indices=[1 3 5]  OutputSizes=1
  Selector6 : Selector  InputPortWidth=12  IndexOptions=Index vector (dialog)  Indices=[7 9 11]  OutputSizes=1
  Selector7 : Selector  InputPortWidth=6  IndexOptions=Index vector (dialog)  Indices=[1 2 3]  OutputSizes=1
  Selector8 : Selector  InputPortWidth=6  IndexOptions=Index vector (dialog)  Indices=[4 5 6]  OutputSizes=1
  Selector9 : Selector  InputPortWidth=12  IndexOptions=Index vector (dialog)  Indices=[2 4 6 8 10 12]  OutputSizes=1
  Subsystem : Subsystem
  Phasors_abc : Outport
  Phasors_Freq : Outport  Port=2
  Phasors_DTFreq : Outport  Port=3
  wires:
  Subsystem/2(Phasors_freq) -> Phasors_Freq/1
  Subsystem/3(Phasors_dtfreq1) -> Phasors_DTFreq/1
  Selector5/1 -> Mux1/1
  Mux1/1 -> Phasors_abc/1
  Selector7/1 -> Mux1/2
  Subsystem/1(Phasors_60Hz) -> Selector5/1, Selector6/1, Selector9/1
  Selector8/1 -> Mux1/4
  Selector6/1 -> Mux1/3
  Measurements/1 -> Subsystem/1(Measurements1)
  Selector9/1 -> Degree to radian1/1(Degree)
  Degree to radian1/1(Radian) -> Selector7/1, Selector8/1

== system feeder_1_3_ss_pmu/SS_PMU/Subsystem5/Subsystem/Subsystem1 ==
  Measurements : Inport
  Degree to radian1 : Subsystem
  Mux1 : Mux
  Selector5 : Selector  InputPortWidth=12  IndexOptions=Index vector (dialog)  Indices=[1 3 5]  OutputSizes=1
  Selector6 : Selector  InputPortWidth=12  IndexOptions=Index vector (dialog)  Indices=[7 9 11]  OutputSizes=1
  Selector7 : Selector  InputPortWidth=6  IndexOptions=Index vector (dialog)  Indices=[1 2 3]  OutputSizes=1
  Selector8 : Selector  InputPortWidth=6  IndexOptions=Index vector (dialog)  Indices=[4 5 6]  OutputSizes=1
  Selector9 : Selector  InputPortWidth=12  IndexOptions=Index vector (dialog)  Indices=[2 4 6 8 10 12]  OutputSizes=1
  Subsystem : Subsystem
  Phasors_abc : Outport
  Phasors_Freq : Outport  Port=2
  Phasors_DTFreq : Outport  Port=3
  wires:
  Subsystem/2(Phasors_freq) -> Phasors_Freq/1
  Subsystem/3(Phasors_dtfreq1) -> Phasors_DTFreq/1
  Selector5/1 -> Mux1/1
  Mux1/1 -> Phasors_abc/1
  Selector7/1 -> Mux1/2
  Subsystem/1(Phasors_60Hz) -> Selector5/1, Selector6/1, Selector9/1
  Selector8/1 -> Mux1/4
  Selector6/1 -> Mux1/3
  Measurements/1 -> Subsystem/1(Measurements1)
  Selector9/1 -> Degree to radian1/1(Degree)
  Degree to radian1/1(Radian) -> Selector7/1, Selector8/1

== system feeder_1_3_ss_pmu/SS_PMU/Subsystem6/Subsystem/Subsystem1 ==
  Measurements : Inport
  Degree to radian1 : Subsystem
  Mux1 : Mux
  Selector5 : Selector  InputPortWidth=12  IndexOptions=Index vector (dialog)  Indices=[1 3 5]  OutputSizes=1
  Selector6 : Selector  InputPortWidth=12  IndexOptions=Index vector (dialog)  Indices=[7 9 11]  OutputSizes=1
  Selector7 : Selector  InputPortWidth=6  IndexOptions=Index vector (dialog)  Indices=[1 2 3]  OutputSizes=1
  Selector8 : Selector  InputPortWidth=6  IndexOptions=Index vector (dialog)  Indices=[4 5 6]  OutputSizes=1
  Selector9 : Selector  InputPortWidth=12  IndexOptions=Index vector (dialog)  Indices=[2 4 6 8 10 12]  OutputSizes=1
  Subsystem : Subsystem
  Phasors_abc : Outport
  Phasors_Freq : Outport  Port=2
  Phasors_DTFreq : Outport  Port=3
  wires:
  Subsystem/2(Phasors_freq) -> Phasors_Freq/1
  Subsystem/3(Phasors_dtfreq1) -> Phasors_DTFreq/1
  Selector5/1 -> Mux1/1
  Mux1/1 -> Phasors_abc/1
  Selector7/1 -> Mux1/2
  Subsystem/1(Phasors_60Hz) -> Selector5/1, Selector6/1, Selector9/1
  Selector8/1 -> Mux1/4
  Selector6/1 -> Mux1/3
  Measurements/1 -> Subsystem/1(Measurements1)
  Selector9/1 -> Degree to radian1/1(Degree)
  Degree to radian1/1(Radian) -> Selector7/1, Selector8/1

== system feeder_1_3_ss_pmu/SS_PMU/Subsystem7/Subsystem/Subsystem1 ==
  Measurements : Inport
  Degree to radian1 : Subsystem
  Mux1 : Mux
  Selector5 : Selector  InputPortWidth=12  IndexOptions=Index vector (dialog)  Indices=[1 3 5]  OutputSizes=1
  Selector6 : Selector  InputPortWidth=12  IndexOptions=Index vector (dialog)  Indices=[7 9 11]  OutputSizes=1
  Selector7 : Selector  InputPortWidth=6  IndexOptions=Index vector (dialog)  Indices=[1 2 3]  OutputSizes=1
  Selector8 : Selector  InputPortWidth=6  IndexOptions=Index vector (dialog)  Indices=[4 5 6]  OutputSizes=1
  Selector9 : Selector  InputPortWidth=12  IndexOptions=Index vector (dialog)  Indices=[2 4 6 8 10 12]  OutputSizes=1
  Subsystem : Subsystem
  Phasors_abc : Outport
  Phasors_Freq : Outport  Port=2
  Phasors_DTFreq : Outport  Port=3
  wires:
  Subsystem/2(Phasors_freq) -> Phasors_Freq/1
  Subsystem/3(Phasors_dtfreq1) -> Phasors_DTFreq/1
  Selector5/1 -> Mux1/1
  Mux1/1 -> Phasors_abc/1
  Selector7/1 -> Mux1/2
  Subsystem/1(Phasors_60Hz) -> Selector5/1, Selector6/1, Selector9/1
  Selector8/1 -> Mux1/4
  Selector6/1 -> Mux1/3
  Measurements/1 -> Subsystem/1(Measurements1)
  Selector9/1 -> Degree to radian1/1(Degree)
  Degree to radian1/1(Radian) -> Selector7/1, Selector8/1

== system feeder_1_3_ss_pmu/SS_PMU/Subsystem8/Subsystem/Subsystem1 ==
  Measurements : Inport
  Degree to radian1 : Subsystem
  Mux1 : Mux
  Selector5 : Selector  InputPortWidth=12  IndexOptions=Index vector (dialog)  Indices=[1 3 5]  OutputSizes=1
  Selector6 : Selector  InputPortWidth=12  IndexOptions=Index vector (dialog)  Indices=[7 9 11]  OutputSizes=1
  Selector7 : Selector  InputPortWidth=6  IndexOptions=Index vector (dialog)  Indices=[1 2 3]  OutputSizes=1
  Selector8 : Selector  InputPortWidth=6  IndexOptions=Index vector (dialog)  Indices=[4 5 6]  OutputSizes=1
  Selector9 : Selector  InputPortWidth=12  IndexOptions=Index vector (dialog)  Indices=[2 4 6 8 10 12]  OutputSizes=1
  Subsystem : Subsystem
  Phasors_abc : Outport
  Phasors_Freq : Outport  Port=2
  Phasors_DTFreq : Outport  Port=3
  wires:
  Subsystem/2(Phasors_freq) -> Phasors_Freq/1
  Subsystem/3(Phasors_dtfreq1) -> Phasors_DTFreq/1
  Selector5/1 -> Mux1/1
  Mux1/1 -> Phasors_abc/1
  Selector7/1 -> Mux1/2
  Subsystem/1(Phasors_60Hz) -> Selector5/1, Selector6/1, Selector9/1
  Selector8/1 -> Mux1/4
  Selector6/1 -> Mux1/3
  Measurements/1 -> Subsystem/1(Measurements1)
  Selector9/1 -> Degree to radian1/1(Degree)
  Degree to radian1/1(Radian) -> Selector7/1, Selector8/1

== system feeder_1_3_ss_pmu/SS_PMU/Subsystem9/Subsystem/Subsystem1 ==
  Measurements : Inport
  Degree to radian1 : Subsystem
  Mux1 : Mux
  Selector5 : Selector  InputPortWidth=12  IndexOptions=Index vector (dialog)  Indices=[1 3 5]  OutputSizes=1
  Selector6 : Selector  InputPortWidth=12  IndexOptions=Index vector (dialog)  Indices=[7 9 11]  OutputSizes=1
  Selector7 : Selector  InputPortWidth=6  IndexOptions=Index vector (dialog)  Indices=[1 2 3]  OutputSizes=1
  Selector8 : Selector  InputPortWidth=6  IndexOptions=Index vector (dialog)  Indices=[4 5 6]  OutputSizes=1
  Selector9 : Selector  InputPortWidth=12  IndexOptions=Index vector (dialog)  Indices=[2 4 6 8 10 12]  OutputSizes=1
  Subsystem : Subsystem
  Phasors_abc : Outport
  Phasors_Freq : Outport  Port=2
  Phasors_DTFreq : Outport  Port=3
  wires:
  Subsystem/2(Phasors_freq) -> Phasors_Freq/1
  Subsystem/3(Phasors_dtfreq1) -> Phasors_DTFreq/1
  Selector5/1 -> Mux1/1
  Mux1/1 -> Phasors_abc/1
  Selector7/1 -> Mux1/2
  Subsystem/1(Phasors_60Hz) -> Selector5/1, Selector6/1, Selector9/1
  Selector8/1 -> Mux1/4
  Selector6/1 -> Mux1/3
  Measurements/1 -> Subsystem/1(Measurements1)
  Selector9/1 -> Degree to radian1/1(Degree)
  Degree to radian1/1(Radian) -> Selector7/1, Selector8/1

== system feeder_1_3_ss_pmu/SS_PMU/zzzOpComm/busStruct/Sub1 ==
  from_signal1 : Inport
  buscre_signal1 : BusCreator  Inputs=17
  demux_signal1 : Demux  Outputs="[6  6  6  6  6  6  6  6  6  6  6  6  6  6  6  6  6]"
  goto_signal1 : Outport
  wires:
  buscre_signal1/1 -> goto_signal1/1  "signal1"
  [rtlab_tag_17] -> buscre_signal1/17  "signal17"
  [rtlab_tag_16] -> buscre_signal1/16  "signal16"
  [rtlab_tag_15] -> buscre_signal1/15  "signal15"
  [rtlab_tag_14] -> buscre_signal1/14  "signal14"
  [rtlab_tag_13] -> buscre_signal1/13  "signal13"
  [rtlab_tag_12] -> buscre_signal1/12  "signal12"
  [rtlab_tag_11] -> buscre_signal1/11  "signal11"
  [rtlab_tag_10] -> buscre_signal1/10  "signal10"
  [rtlab_tag_9] -> buscre_signal1/9  "signal9"
  [rtlab_tag_8] -> buscre_signal1/8  "signal8"
  [rtlab_tag_7] -> buscre_signal1/7  "signal7"
  [rtlab_tag_6] -> buscre_signal1/6  "signal6"
  [rtlab_tag_5] -> buscre_signal1/5  "signal5"
  [rtlab_tag_4] -> buscre_signal1/4  "signal4"
  [rtlab_tag_3] -> buscre_signal1/3  "signal3"
  [rtlab_tag_2] -> buscre_signal1/2  "signal2"
  [rtlab_tag_1] -> buscre_signal1/1  "signal1"
  demux_signal1/17 -> [rtlab_tag_17]
  demux_signal1/16 -> [rtlab_tag_16]
  demux_signal1/15 -> [rtlab_tag_15]
  demux_signal1/14 -> [rtlab_tag_14]
  demux_signal1/13 -> [rtlab_tag_13]
  demux_signal1/12 -> [rtlab_tag_12]
  demux_signal1/11 -> [rtlab_tag_11]
  demux_signal1/10 -> [rtlab_tag_10]
  demux_signal1/9 -> [rtlab_tag_9]
  demux_signal1/8 -> [rtlab_tag_8]
  demux_signal1/7 -> [rtlab_tag_7]
  demux_signal1/6 -> [rtlab_tag_6]
  demux_signal1/5 -> [rtlab_tag_5]
  demux_signal1/4 -> [rtlab_tag_4]
  demux_signal1/3 -> [rtlab_tag_3]
  demux_signal1/2 -> [rtlab_tag_2]
  demux_signal1/1 -> [rtlab_tag_1]
  from_signal1/1 -> demux_signal1/1

== system feeder_1_3_ss_pmu/SS_PMU/zzzOpComm/busStruct/Sub2 ==
  in : Inport
  out : Outport
  wires:
  in/1 -> out/1  "signal1"

== system feeder_1_3_ss_pmu/SS_PMU/zzzOpComm/busStruct/Sub3 ==
  in : Inport
  out : Outport
  wires:
  in/1 -> out/1  "signal1"

== system feeder_1_3_ss_pmu/SS_PMU/Subsystem1/Subsystem/Subsystem1/Degree to radian1 ==
  Degree : Inport
  Constant : Constant  Value=pi
  Constant1 : Constant  Value=180
  Divide : Product  Inputs=*/
  Product : Product  RndMeth=Zero
  Radian : Outport
  wires:
  Divide/1 -> Radian/1
  Degree/1 -> Product/1
  Constant1/1 -> Divide/2
  Product/1 -> Divide/1
  Constant/1 -> Product/2

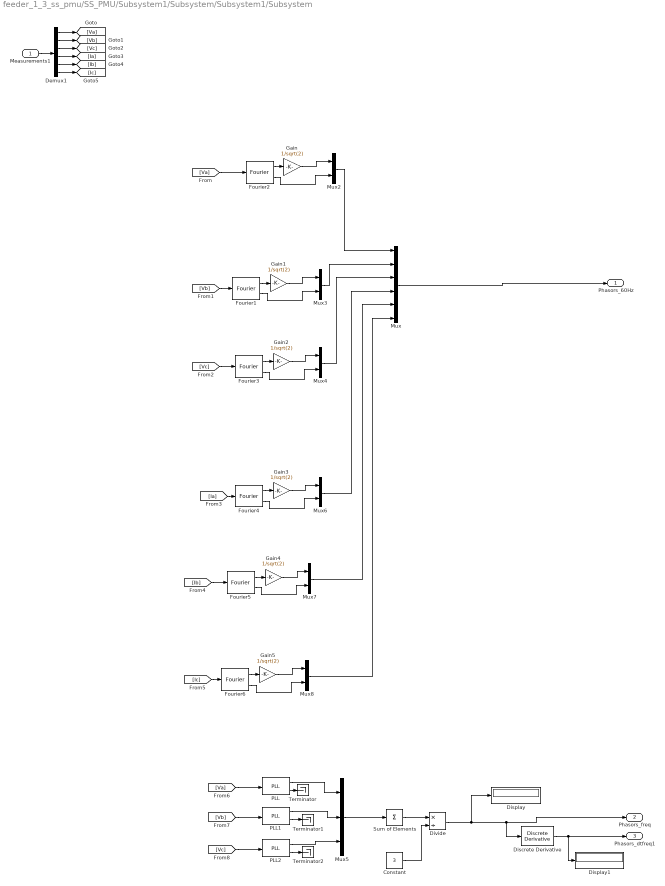
== system feeder_1_3_ss_pmu/SS_PMU/Subsystem1/Subsystem/Subsystem1/Subsystem ==
  Measurements1 : Inport
  Constant : Constant  Value=3
  Demux1 : Demux  Outputs=6
  Discrete Derivative : simulink/Discrete/Discrete Derivative  gainval=1.0  ICPrevScaledInput=0.0  OutMin=[]  OutMax=[]  OutDataType=fixdt(1, 16)  OutScaling=2^-10  DoSatur=off
  Display : Display
  Display1 : Display
  Divide : Product  Inputs=*/
  Fourier{1..6} (6 alike) : powerlib_meascontrol/Measurements/Fourier  Freq=60  n=1  InInit=[0, 0]  Ts=Ts
      settings: SourceProductName=Simscape Power Systems
  Gain{,1..5} (6 alike) : Gain  Gain=1/sqrt(2)
  Mux : Mux  Inputs=6
  Mux{2..4,6..8} (6 alike) : Mux  Inputs=2
  Mux5 : Mux  Inputs=3
  PLL : powerlib_meascontrol/PLL/PLL  Fmin=60  Par_Init=[0, 60]  ParK=[180, 3200, 1]  TcD=1.6e-4  MaxRateChangeFreq=12  FilterCutOffFreq=25  Ts=Ts  AGC=on
      settings: SourceProductName=Simscape Power Systems  SourceProductBaseCode=PS
  PLL1 : powerlib_meascontrol/PLL/PLL  Fmin=60  Par_Init=[0, 60]  ParK=[180, 3200, 1]  TcD=1.6e-4  MaxRateChangeFreq=12  FilterCutOffFreq=25  Ts=Ts  AGC=on
      settings: SourceProductName=Simscape Power Systems  SourceProductBaseCode=PS
  PLL2 : powerlib_meascontrol/PLL/PLL  Fmin=60  Par_Init=[0, 60]  ParK=[180, 3200, 1]  TcD=1.6e-4  MaxRateChangeFreq=12  FilterCutOffFreq=25  Ts=Ts  AGC=on
      settings: SourceProductName=Simscape Power Systems  SourceProductBaseCode=PS
  Sum of Elements : Sum  Inputs=+
  Terminator : Terminator
  Terminator1 : Terminator
  Terminator2 : Terminator
  Phasors_60Hz : Outport
  Phasors_freq : Outport  Port=2
  Phasors_dtfreq1 : Outport  Port=3
  wires:
  Mux5/1 -> Sum of Elements/1
  PLL2/1 -> Mux5/3
  PLL1/1 -> Mux5/2
  PLL/1 -> Mux5/1
  PLL2/2 -> Terminator2/1
  PLL1/2 -> Terminator1/1
  PLL/2 -> Terminator/1
  [Vc] -> PLL2/1
  [Vb] -> PLL1/1
  [Va] -> PLL/1
  Discrete Derivative/1 -> Display1/1, Phasors_dtfreq1/1
  Mux3/1 -> Mux/2
  Mux2/1 -> Mux/1
  Demux1/2 -> [Vb]
  Measurements1/1 -> Demux1/1
  [Va] -> Fourier2/1
  Demux1/3 -> [Vc]
  Demux1/1 -> [Va]
  Mux7/1 -> Mux/5
  Mux4/1 -> Mux/3
  Mux/1 -> Phasors_60Hz/1
  Demux1/4 -> [Ia]
  Demux1/6 -> [Ic]
  Demux1/5 -> [Ib]
  Mux8/1 -> Mux/6
  Mux6/1 -> Mux/4
  Sum of Elements/1 -> Divide/1
  Divide/1 -> Display/1, Discrete Derivative/1, Phasors_freq/1
  Constant/1 -> Divide/2
  Fourier2/2 -> Mux2/2
  [Vc] -> Fourier3/1
  [Ia] -> Fourier4/1
  Fourier2/1 -> Gain/1
  Gain/1 -> Mux2/1
  [Vb] -> Fourier1/1
  Fourier1/2 -> Mux3/2
  Fourier1/1 -> Gain1/1
  Gain1/1 -> Mux3/1
  Fourier3/2 -> Mux4/2
  Fourier3/1 -> Gain2/1
  Gain2/1 -> Mux4/1
  Fourier4/2 -> Mux6/2
  Fourier4/1 -> Gain3/1
  Gain3/1 -> Mux6/1
  Fourier5/2 -> Mux7/2
  Fourier5/1 -> Gain4/1
  Gain4/1 -> Mux7/1
  Fourier6/2 -> Mux8/2
  Fourier6/1 -> Gain5/1
  Gain5/1 -> Mux8/1
  [Ic] -> Fourier6/1
  [Ib] -> Fourier5/1

== system feeder_1_3_ss_pmu/SS_PMU/Subsystem10/Subsystem/Subsystem1/Degree to radian1 ==
  Degree : Inport
  Constant : Constant  Value=pi
  Constant1 : Constant  Value=180
  Divide : Product  Inputs=*/
  Product : Product  RndMeth=Zero
  Radian : Outport
  wires:
  Divide/1 -> Radian/1
  Degree/1 -> Product/1
  Constant1/1 -> Divide/2
  Product/1 -> Divide/1
  Constant/1 -> Product/2
